simulink model "dspvorbisdec"  (Simulink 8.3)
settings: Solver=FixedStepDiscrete  SolverMode=SingleTasking  StartTime=0.0  StopTime=inf  RelTol=1e-3
model workspace (MAT data in the model file):
  oggData = [79 103 103 83 0 2 0 0 0 0 0 0 ... (70501 elements, 70501x1)]
  dspvorbisdec_OutputSampRt : num (value not decoded)
PostLoadFcn:
  | hws  = get_param(bdroot,'modelworkspace');
  | dspvorbisdec_SampRt = hws.evalin('dspvorbisdec_OutputSampRt');
  | clear hws;
StopFcn:
  | dspvorbisdec_hws = get_param(bdroot,'modelworkspace');
  | dspvorbisdec_tmp = dspvorbisdec_hws.data;
  | for i = 1:length(dspvorbisdec_tmp)
  |   if strcmp(dspvorbisdec_tmp(i).Name,'dspvorbisdec_OutputSampRt')
  |      if (dspvorbisdec_tmp(i).Value~=dspvorbisdec_SampRt)
  |         dspvorbisdec_hws.assignin('dspvorbisdec_OutputSampRt', dspvorbisdec_SampRt);
  |      end
  |   end
  | end
  | 
  | clear hws dspvorbisdec_tmp i dspvorbisdec_hws;
undefined symbols (not defined in the file or in its folder): blockSize, errordlg, uiwait, warndlg
libraries: simulink x5, dspmtrx3 x3, dspindex x2, dspsigops x1, dspxfrm3 x1, dspmisc x1, dspsnks4 x1, dspsrcs4 x1
(part 1 of 3)
CloseFcn:
  | clear dspvorbisdec_SampRt;
settings Model: FPTRunName=Active  Creator=The MathWorks Inc.  ExtModeAutoUpdateStatusClock=off
settings DataIOCC: SaveOutput=off  SignalLogging=off  SaveTime=off
settings OptimizationCC: InlineParams=on  ExpressionDepthLimit=2147483647  InitFltsAndDblsToZero=on  EfficientMapNaN2IntZero=off
settings DebuggingCC: SaveWithParameterizedLinksMsg=none  MultiTaskDSMMsg=warning  MultiTaskCondExecSysMsg=none  FcnCallInpInsideContextMsg=UseLocalSettings  StrictBusMsg=Warning
settings HardwareCC: TargetBitPerLong=64  TargetBitPerPointer=64  TargetLongLongMode=on  TargetEndianess=LittleEndian  TargetWordSize=64  TargetHWDeviceType=MATLAB Host  ProdEqTarget=off
settings SFSimCC: SFSimEnableDebug=off  SFSimOverflowDetection=off  SFSimEcho=off  SimParseCustomCode=off
settings GRTTargetCC: TargetFcnLib=ansi_tfl_tmw.mat

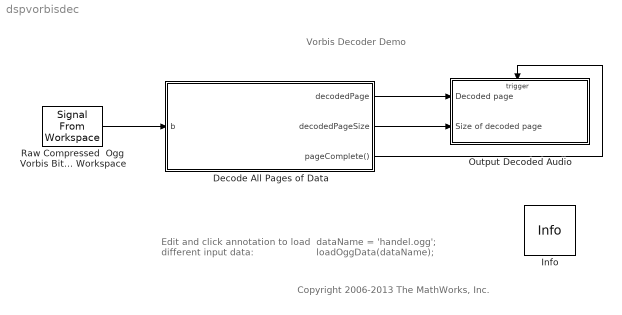
== system dspvorbisdec ==
  note: Vorbis Decoder Demo
  note: Copyright 2006-2013 The MathWorks, Inc.
  note: dataName = 'handel.ogg';
      | loadOggData(dataName);
  note: Edit and click annotation to
      | load different input data:
  Decode All Pages of Data : Stateflow chart  TreatAsAtomicUnit=on
  Info : dspmisc/Info  SystemSampleTime=-1
  Output Decoded Audio : Subsystem  TreatAsAtomicUnit=on
  Raw Compressed  Ogg Vorbis Bitstream  from Workspace : dspsrcs4/Signal From Workspace  X=oggData  Ts=1  nsamps=1  OutputAfterFinalValue=Cyclic repetition  ignoreOrWarnInputAndFrameLengths=off
  wires:
  Raw Compressed  Ogg Vorbis Bitstream  from Workspace/1 -> Decode All Pages of Data/1(b)
  Decode All Pages of Data/3(pageComplete()) -> Output Decoded Audio/Trigger
  Decode All Pages of Data/1(decodedPage) -> Output Decoded Audio/1(Decoded page)
  Decode All Pages of Data/2(decodedPageSize) -> Output Decoded Audio/2(Size of decoded page)

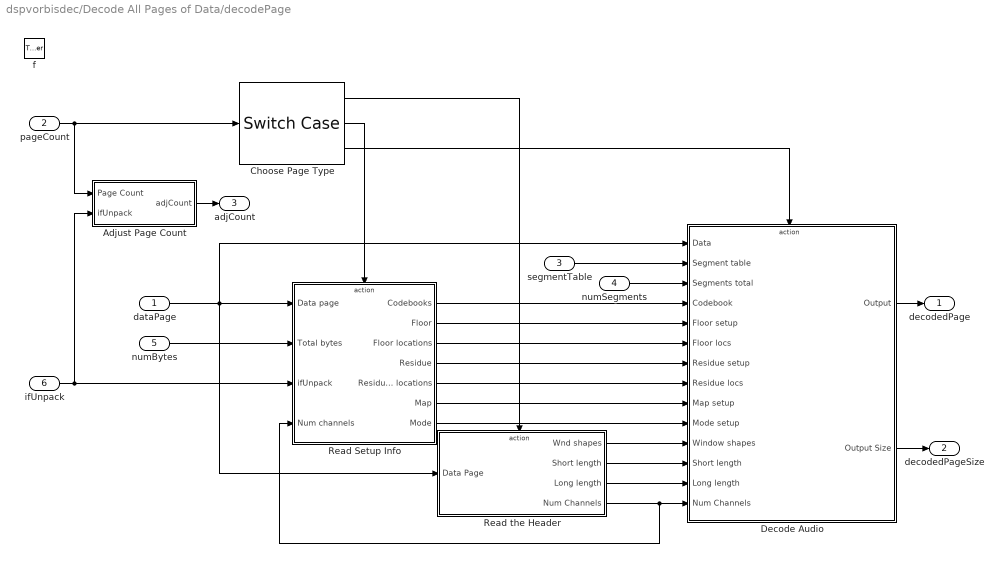
== system dspvorbisdec/Decode All Pages of Data/decodePage ==
  dataPage : Inport  OutDataTypeStr=uint8  PortDimensions=5500
  pageCount : Inport  Port=2  OutDataTypeStr=uint16  PortDimensions=1
  segmentTable : Inport  Port=3  OutDataTypeStr=uint16  PortDimensions=255
  numSegments : Inport  Port=4  OutDataTypeStr=uint16  PortDimensions=1
  numBytes : Inport  Port=5  OutDataTypeStr=uint16  PortDimensions=1
  ifUnpack : Inport  Port=6  OutDataTypeStr=boolean  PortDimensions=1
  f : TriggerPort  TriggerType=function-call
      settings: CopyFcn=Stateflow.SLINSF.SimulinkMan.removeBlockPreDeleteFcn  PreDeleteFcn=Stateflow.SLINSF.SimulinkMan.unsafePredeleteFcn
  Adjust Page Count : Subsystem
  Choose Page Type : SwitchCase  CaseConditions={1, 2}
  Decode Audio : Subsystem  TreatAsAtomicUnit=on
  Read Setup Info : Subsystem  TreatAsAtomicUnit=on
  Read the Header : Subsystem  TreatAsAtomicUnit=on
  decodedPage : Outport
  decodedPageSize : Outport  Port=2  OutputWhenDisabled=reset  InitialOutput=0
  adjCount : Outport  Port=3  OutputWhenDisabled=reset  InitialOutput=0
  wires:
  dataPage/1 -> Read the Header/1(Data Page), Decode Audio/1(Data), Read Setup Info/1(Data page)
  pageCount/1 -> Choose Page Type/1, Adjust Page Count/1(Page Count)
  Choose Page Type/1 -> Read the Header/Action
  Choose Page Type/2 -> Read Setup Info/Action
  numBytes/1 -> Read Setup Info/2(Total bytes)
  Read Setup Info/7(Mode) -> Decode Audio/10(Mode setup)
  Read Setup Info/6(Map) -> Decode Audio/9(Map setup)
  Read Setup Info/5(Residue locations) -> Decode Audio/8(Residue locs)
  Read Setup Info/4(Residue) -> Decode Audio/7(Residue setup)
  Read Setup Info/3(Floor locations) -> Decode Audio/6(Floor locs)
  Read Setup Info/2(Floor) -> Decode Audio/5(Floor setup)
  Read Setup Info/1(Codebooks) -> Decode Audio/4(Codebook)
  numSegments/1 -> Decode Audio/3(Segments total)
  segmentTable/1 -> Decode Audio/2(Segment table)
  Read the Header/1(Wnd shapes) -> Decode Audio/11(Window shapes)
  Read the Header/4(Num Channels) -> Decode Audio/14(Num Channels), Read Setup Info/4(Num channels)
  Read the Header/3(Long length) -> Decode Audio/13(Long length)
  Read the Header/2(Short length) -> Decode Audio/12(Short length)
  Decode Audio/1(Output) -> decodedPage/1
  Decode Audio/2(Output Size) -> decodedPageSize/1
  Choose Page Type/3 -> Decode Audio/Action
  ifUnpack/1 -> Read Setup Info/3(ifUnpack), Adjust Page Count/2(ifUnpack)
  Adjust Page Count/1(adjCount) -> adjCount/1

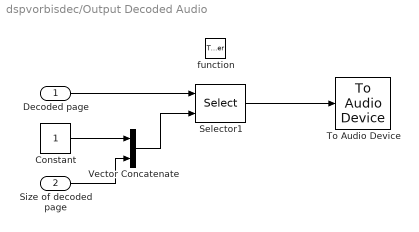
== system dspvorbisdec/Output Decoded Audio ==
  Decoded page : Inport
  Size of decoded page : Inport  Port=2
  function : TriggerPort  TriggerType=function-call
  Constant : Constant  OutDataTypeStr=int32
  Selector1 : Selector  NumberOfDimensions=2  IndexMode=Zero-based  InputPortWidth=3  IndexOptions=Starting and ending indices (port),Select all  Indices=[1 3],1  OutputSizes=32,1
  To Audio Device : dspsnks4/To Audio Device  deviceName=Default  inheritSampleRate=off  sampleRate=dspvorbisdec_OutputSampRt  deviceDatatype=Determine from input data type  autoBufferSize=on  bufferSize=1024  queueDuration=1  defaultOutputChannelMapping=on  outputChannelMapping=1
  Vector Concatenate : Concatenate
  wires:
  Size of decoded page/1 -> Vector Concatenate/2
  Selector1/1 -> To Audio Device/1
  Constant/1 -> Vector Concatenate/1
  Vector Concatenate/1 -> Selector1/2
  Decoded page/1 -> Selector1/1

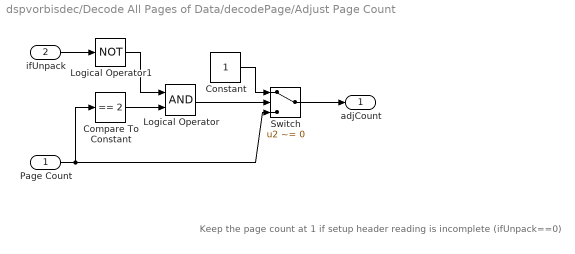
== system dspvorbisdec/Decode All Pages of Data/decodePage/Adjust Page Count ==
  note: Keep the page count at 1 if setup header reading is incomplete (ifUnpack==0)
  Page Count : Inport
  ifUnpack : Inport  Port=2
  Compare To Constant : simulink/Logic and Bit Operations/Compare To Constant  relop===  const=2  OutDataTypeStr=boolean  ZeroCross=off
  Constant : Constant  OutDataTypeStr=uint16
  Logical Operator : Logic  AllPortsSameDT=off  OutDataTypeStr=boolean
  Logical Operator1 : Logic  Operator=NOT  AllPortsSameDT=off  OutDataTypeStr=boolean
  Switch : Switch  Criteria=u2 ~= 0
  adjCount : Outport
  wires:
  Logical Operator/1 -> Switch/2
  Constant/1 -> Switch/1
  Page Count/1 -> Switch/3, Compare To Constant/1
  ifUnpack/1 -> Logical Operator1/1
  Logical Operator1/1 -> Logical Operator/1
  Compare To Constant/1 -> Logical Operator/2
  Switch/1 -> adjCount/1

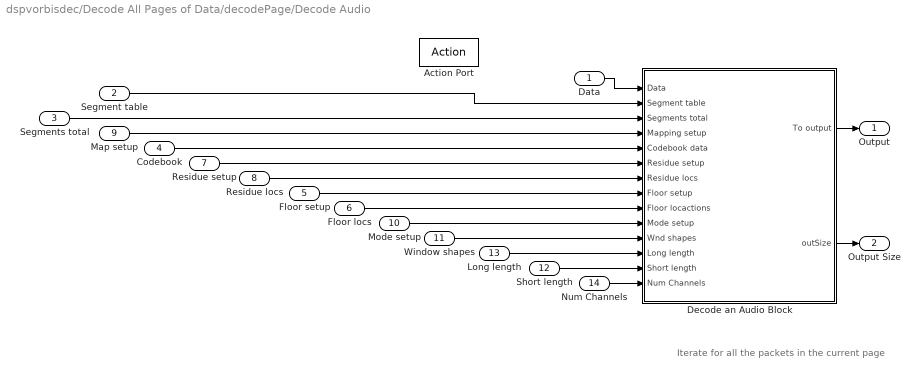
== system dspvorbisdec/Decode All Pages of Data/decodePage/Decode Audio ==
  note: Iterate for all the packets in the current page
  Data : Inport
  Segment table : Inport  Port=2
  Segments total : Inport  Port=3
  Codebook : Inport  Port=4
  Floor setup : Inport  Port=5
  Floor locs : Inport  Port=6
  Residue setup : Inport  Port=7
  Residue locs : Inport  Port=8
  Map setup : Inport  Port=9
  Mode setup : Inport  Port=10
  Window shapes : Inport  Port=11
  Short length : Inport  Port=12
  Long length : Inport  Port=13
  Num Channels : Inport  Port=14
  Action Port : ActionPort  PropagateVarSize=During execution  ActionType=default
  Decode an Audio Block : Subsystem  TreatAsAtomicUnit=on
  Output : Outport
  Output Size : Outport  Port=2  OutputWhenDisabled=reset  InitialOutput=0
  wires:
  Segment table/1 -> Decode an Audio Block/2(Segment table)
  Segments total/1 -> Decode an Audio Block/3(Segments total)
  Map setup/1 -> Decode an Audio Block/4(Mapping setup)
  Codebook/1 -> Decode an Audio Block/5(Codebook data)
  Residue setup/1 -> Decode an Audio Block/6(Residue setup)
  Residue locs/1 -> Decode an Audio Block/7(Residue locs)
  Floor setup/1 -> Decode an Audio Block/8(Floor setup)
  Floor locs/1 -> Decode an Audio Block/9(Floor locactions)
  Mode setup/1 -> Decode an Audio Block/10(Mode setup)
  Window shapes/1 -> Decode an Audio Block/11(Wnd shapes)
  Long length/1 -> Decode an Audio Block/12(Long length)
  Short length/1 -> Decode an Audio Block/13(Short length)
  Decode an Audio Block/1(To output) -> Output/1
  Decode an Audio Block/2(outSize) -> Output Size/1
  Num Channels/1 -> Decode an Audio Block/14(Num Channels)
  Data/1 -> Decode an Audio Block/1(Data)

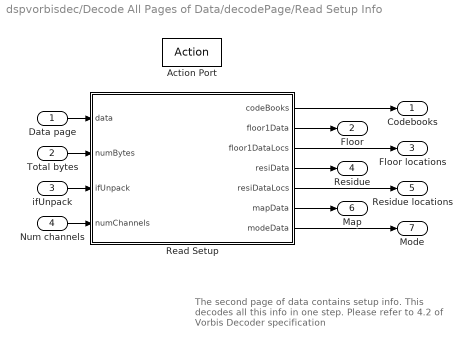
== system dspvorbisdec/Decode All Pages of Data/decodePage/Read Setup Info ==
  note: The second page of data contains
      | setup info. This decodes all this info in one step.
      | Please refer to 4.2 of Vorbis Decoder specification
  Data page : Inport
  Total bytes : Inport  Port=2
  ifUnpack : Inport  Port=3
  Num channels : Inport  Port=4
  Action Port : ActionPort  PropagateVarSize=During execution  ActionType=case
  Read Setup : MATLAB Function  TreatAsAtomicUnit=on
  Codebooks : Outport
  Floor : Outport  Port=2
  Floor locations : Outport  Port=3
  Residue : Outport  Port=4
  Residue locations : Outport  Port=5
  Map : Outport  Port=6
  Mode : Outport  Port=7
  wires:
  Data page/1 -> Read Setup/1(data)
  Total bytes/1 -> Read Setup/2(numBytes)
  Read Setup/1(codeBooks) -> Codebooks/1
  Read Setup/2(floor1Data) -> Floor/1
  Read Setup/3(floor1DataLocs) -> Floor locations/1
  Read Setup/4(resiData) -> Residue/1
  Read Setup/5(resiDataLocs) -> Residue locations/1
  Read Setup/6(mapData) -> Map/1
  Read Setup/7(modeData) -> Mode/1
  Num channels/1 -> Read Setup/4(numChannels)
  ifUnpack/1 -> Read Setup/3(ifUnpack)

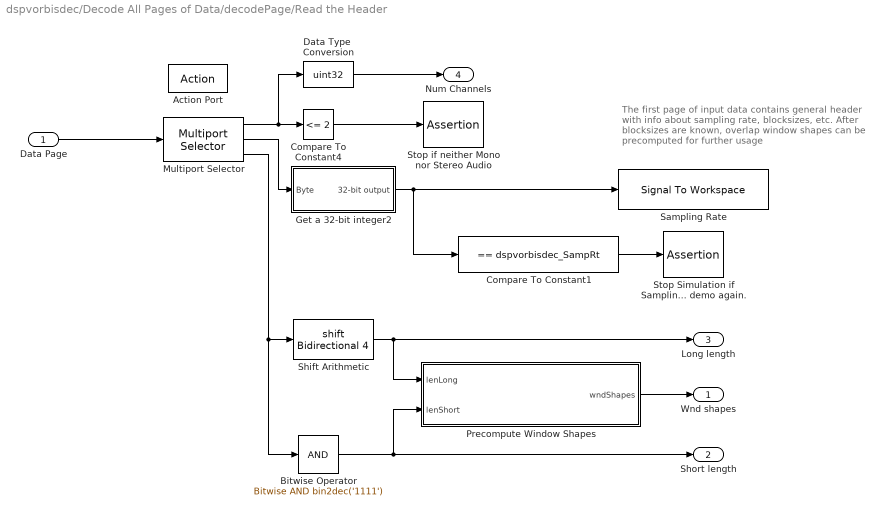
== system dspvorbisdec/Decode All Pages of Data/decodePage/Read the Header ==
  note: The first page of input data contains general header
      | with info about sampling rate, blocksizes, etc.
      | After blocksizes are known, overlap window shapes
      | can be precomputed for further usage
  Data Page : Inport
  Action Port : ActionPort  PropagateVarSize=During execution  ActionType=case
  Bitwise Operator : simulink/Logic and Bit Operations/Bitwise Operator  logicop=AND  UseBitMask=on  BitMask=bin2dec('1111')  BitMaskRealWorld=Stored Integer
  Compare To Constant1 : simulink/Logic and Bit Operations/Compare To Constant  relop===  const=dspvorbisdec_SampRt  OutDataTypeStr=boolean  ZeroCross=off
  Compare To Constant4 : simulink/Logic and Bit Operations/Compare To Constant  relop=<=  const=2  OutDataTypeStr=boolean  ZeroCross=off
  Data Type  Conversion : DataTypeConversion  OutDataTypeStr=uint32  SaturateOnIntegerOverflow=on  RndMeth=Zero
  Get a 32-bit integer2 : Subsystem
  Multiport Selector : dspindex/Multiport Selector  rowsOrCols=Rows  idxCellArray={12, 13:16, 29}  idxErrMode=Clip Index
  Precompute Window Shapes : MATLAB Function  TreatAsAtomicUnit=on
  Sampling Rate : SignalToWorkspace  VariableName=dspvorbisdec_SampRt
      settings: CopyFcn=dspblkcopystw(gcbh);  MaxDataPoints=1  Save2DSignal=3-D array (concatenate along third dimension)
  Shift Arithmetic : ArithShift  BitShiftNumber=4
  Stop Simulation if Sampling Rate is Different Than Before. Run the demo again. : Assertion  AssertionFailFcn=uiwait(warndlg('Output the sampling rate has been updated. Please stop the simulation and run the demo again.','DSP System Toolbox Demo Warning','modal'));  StopWhenAssertionFail=off
  Stop if neither Mono nor Stereo Audio : Assertion  AssertionFailFcn=uiwait(errordlg('This demo only supports monophonic or stereo audio inputs.','DSP System Toolbox Demo Error','modal'));
  Wnd shapes : Outport
  Short length : Outport  Port=2
  Long length : Outport  Port=3
  Num Channels : Outport  Port=4
  wires:
  Data Page/1 -> Multiport Selector/1
  Multiport Selector/1 -> Compare To Constant4/1, Data Type  Conversion/1
  Multiport Selector/2 -> Get a 32-bit integer2/1(Byte)
  Get a 32-bit integer2/1(32-bit output) -> Sampling Rate/1, Compare To Constant1/1
  Bitwise Operator/1 -> Precompute Window Shapes/2(lenShort), Short length/1
  Shift Arithmetic/1 -> Precompute Window Shapes/1(lenLong), Long length/1
  Precompute Window Shapes/1(wndShapes) -> Wnd shapes/1
  Multiport Selector/3 -> Shift Arithmetic/1, Bitwise Operator/1
  Compare To Constant4/1 -> Stop if neither Mono nor Stereo Audio/1
  Data Type  Conversion/1 -> Num Channels/1
  Compare To Constant1/1 -> Stop Simulation if Sampling Rate is Different Than Before. Run the demo again./1

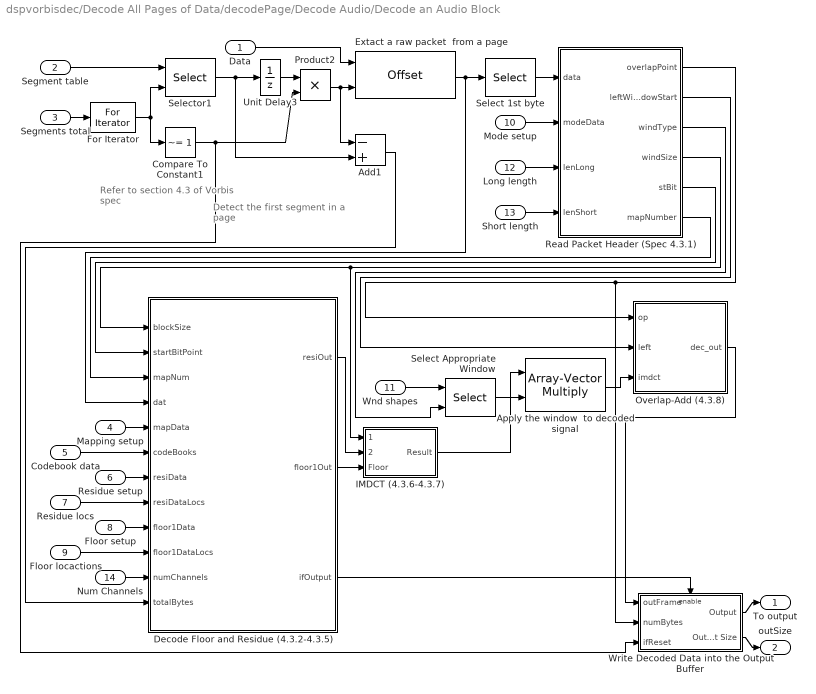
== system dspvorbisdec/Decode All Pages of Data/decodePage/Decode Audio/Decode an Audio Block ==
  note: Refer to section 4.3 of
      | Vorbis spec
  note: Detect the first
      | segment in a page
  Data : Inport
  Segment table : Inport  Port=2
  Segments total : Inport  Port=3
  Mapping setup : Inport  Port=4
  Codebook data : Inport  Port=5
  Residue setup : Inport  Port=6
  Residue locs : Inport  Port=7
  Floor setup : Inport  Port=8
  Floor locactions : Inport  Port=9
  Mode setup : Inport  Port=10
  Wnd shapes : Inport  Port=11
  Long length : Inport  Port=12
  Short length : Inport  Port=13
  Num Channels : Inport  Port=14
  Add1 : Sum  Inputs=-+
  Apply the window  to decoded signal : dspmtrx3/Array-Vector Multiply  mode=Mute  saveAsFlag=0  Dimension=1  V_Source=Input port  V_VectFromMask=[0.5 0.25]  firstCoeffSignedness=Auto  firstCoeffDataTypeStr=Inherit: Same word length as input  firstCoeffLastDataTypeStr=Inherit: Same word length as input  firstCoeffMin=[]  firstCoeffMax=[]  outputSignedness=Auto  outputDataTypeStr=Inherit: Same as product output  outputLastDataTypeStr=Inherit: Same as product output  outputMin=[]  outputMax=[]  accumSignedness=Auto  prodOutputSignedness=Auto  roundingMode=Floor  overflowMode=off
  Compare To Constant1 : simulink/Logic and Bit Operations/Compare To Constant  relop=~=  const=1  OutDataTypeStr=uint8  ZeroCross=off
  Decode Floor and Residue (4.3.2-4.3.5) : MATLAB Function  TreatAsAtomicUnit=on
  Extact a raw packet  from a page : dspsigops/Offset  mode=Remove beginning samples  numDatOffPair=1  outWidthSpec=User-defined  outWidth=2048  actionOutRange=Clip
  For Iterator : ForIterator  IterationSource=external
  IMDCT (4.3.6-4.3.7) : Subsystem
  Overlap-Add (4.3.8) : Subsystem
  Product2 : Product  OutDataTypeStr=uint16  RndMeth=Zero
  Read Packet Header (Spec 4.3.1) : MATLAB Function  TreatAsAtomicUnit=on
  Select 1st byte : Selector  InputPortWidth=2048  Indices=[1]
  Select Appropriate Window : Selector  NumberOfDimensions=2  InputPortWidth=8192  IndexOptions=Select all,Index vector (port)  Indices=1,-1
  Selector1 : Selector  InputPortWidth=255  IndexOptions=Index vector (port)  Indices=[1 3]
  Unit Delay3 : UnitDelay  SampleTime=-1
  Write Decoded Data into the Output Buffer : Subsystem  TreatAsAtomicUnit=on
  To output : Outport
  outSize : Outport  Port=2
  wires:
  Segments total/1 -> For Iterator/1
  Segment table/1 -> Selector1/1
  Unit Delay3/1 -> Product2/1
  Compare To Constant1/1 -> Product2/2, Write Decoded Data into the Output Buffer/3(ifReset)
  For Iterator/1 -> Selector1/2, Compare To Constant1/1
  Mode setup/1 -> Read Packet Header (Spec 4.3.1)/2(modeData)
  Long length/1 -> Read Packet Header (Spec 4.3.1)/3(lenLong)
  Short length/1 -> Read Packet Header (Spec 4.3.1)/4(lenShort)
  Mapping setup/1 -> Decode Floor and Residue (4.3.2-4.3.5)/5(mapData)
  Codebook data/1 -> Decode Floor and Residue (4.3.2-4.3.5)/6(codeBooks)
  Residue setup/1 -> Decode Floor and Residue (4.3.2-4.3.5)/7(resiData)
  Residue locs/1 -> Decode Floor and Residue (4.3.2-4.3.5)/8(resiDataLocs)
  Floor setup/1 -> Decode Floor and Residue (4.3.2-4.3.5)/9(floor1Data)
  Floor locactions/1 -> Decode Floor and Residue (4.3.2-4.3.5)/10(floor1DataLocs)
  Read Packet Header (Spec 4.3.1)/5(stBit) -> Decode Floor and Residue (4.3.2-4.3.5)/2(startBitPoint)
  Read Packet Header (Spec 4.3.1)/6(mapNumber) -> Decode Floor and Residue (4.3.2-4.3.5)/3(mapNum)
  Decode Floor and Residue (4.3.2-4.3.5)/2(floor1Out) -> IMDCT (4.3.6-4.3.7)/3(Floor)
  Read Packet Header (Spec 4.3.1)/4(windSize) -> Decode Floor and Residue (4.3.2-4.3.5)/1(blockSize), IMDCT (4.3.6-4.3.7)/1(Wnd len)
  Read Packet Header (Spec 4.3.1)/3(windType) -> Select Appropriate Window/2
  Read Packet Header (Spec 4.3.1)/2(leftWindowStart) -> Overlap-Add (4.3.8)/2(left)
  Read Packet Header (Spec 4.3.1)/1(overlapPoint) -> Write Decoded Data into the Output Buffer/2(numBytes), Overlap-Add (4.3.8)/1(op)
  Extact a raw packet  from a page/1 -> Select 1st byte/1, Decode Floor and Residue (4.3.2-4.3.5)/4(dat)
  Select 1st byte/1 -> Read Packet Header (Spec 4.3.1)/1(data)
  Product2/1 -> Extact a raw packet  from a page/2, Add1/1
  Data/1 -> Extact a raw packet  from a page/1
  Num Channels/1 -> Decode Floor and Residue (4.3.2-4.3.5)/11(numChannels)
  IMDCT (4.3.6-4.3.7)/1(Result) -> Apply the window  to decoded signal/1
  Add1/1 -> Decode Floor and Residue (4.3.2-4.3.5)/12(totalBytes)
  Selector1/1 -> Unit Delay3/1, Add1/2
  Write Decoded Data into the Output Buffer/1(Output) -> To output/1
  Decode Floor and Residue (4.3.2-4.3.5)/1(resiOut) -> IMDCT (4.3.6-4.3.7)/2(Residue)
  Decode Floor and Residue (4.3.2-4.3.5)/3(ifOutput) -> Write Decoded Data into the Output Buffer/Enable
  Wnd shapes/1 -> Select Appropriate Window/1
  Select Appropriate Window/1 -> Apply the window  to decoded signal/2
  Apply the window  to decoded signal/1 -> Overlap-Add (4.3.8)/3(imdct)
  Overlap-Add (4.3.8)/1(dec_out) -> Write Decoded Data into the Output Buffer/1(outFrame)
  Write Decoded Data into the Output Buffer/2(Output Size) -> outSize/1

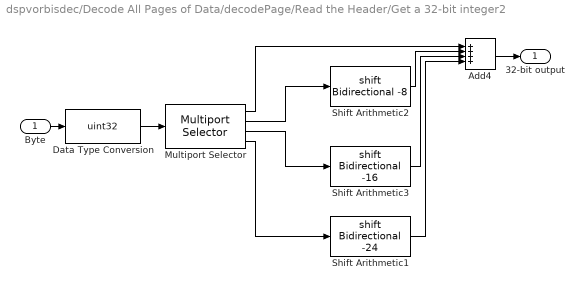
== system dspvorbisdec/Decode All Pages of Data/decodePage/Read the Header/Get a 32-bit integer2 ==
  Byte : Inport
  Add4 : Sum  Inputs=++++
  Data Type Conversion : DataTypeConversion  OutDataTypeStr=uint32  ConvertRealWorld=Stored Integer (SI)
  Multiport Selector : dspindex/Multiport Selector  rowsOrCols=Rows  idxCellArray={ 1,2,3,4 }  idxErrMode=Clip Index
  Shift Arithmetic1 : ArithShift  BitShiftNumber=-24
  Shift Arithmetic2 : ArithShift  BitShiftNumber=-8
  Shift Arithmetic3 : ArithShift  BitShiftNumber=-16
  32-bit output : Outport
  wires:
  Multiport Selector/4 -> Shift Arithmetic1/1
  Multiport Selector/1 -> Add4/1
  Data Type Conversion/1 -> Multiport Selector/1
  Multiport Selector/2 -> Shift Arithmetic2/1
  Multiport Selector/3 -> Shift Arithmetic3/1
  Add4/1 -> 32-bit output/1
  Byte/1 -> Data Type Conversion/1
  Shift Arithmetic3/1 -> Add4/3
  Shift Arithmetic2/1 -> Add4/2
  Shift Arithmetic1/1 -> Add4/4

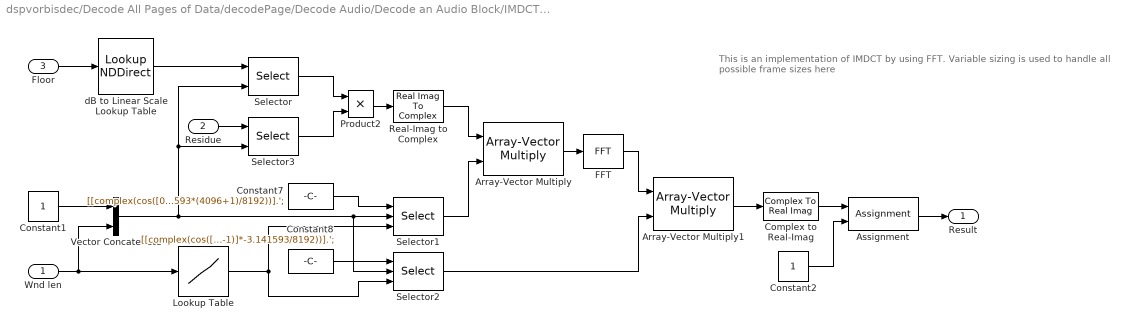
== system dspvorbisdec/Decode All Pages of Data/decodePage/Decode Audio/Decode an Audio Block/IMDCT (4.3.6-4.3.7) ==
  note: This is an implementation of IMDCT by using FFT.
      | Variable sizing is used to handle all possible frame sizes here
  Wnd len : Inport
  Residue : Inport  Port=2
  Floor : Inport  Port=3
  Array-Vector Multiply : dspmtrx3/Array-Vector Multiply  mode=Mute  saveAsFlag=0  Dimension=1  V_Source=Input port  V_VectFromMask=[0.5 0.25]  firstCoeffSignedness=Auto  firstCoeffDataTypeStr=Inherit: Same word length as input  firstCoeffLastDataTypeStr=Inherit: Same word length as input  firstCoeffMin=[]  firstCoeffMax=[]  outputSignedness=Auto  outputDataTypeStr=Inherit: Same as product output  outputLastDataTypeStr=Inherit: Same as product output  outputMin=[]  outputMax=[]  accumSignedness=Auto  prodOutputSignedness=Auto  roundingMode=Floor  overflowMode=off
  Array-Vector Multiply1 : dspmtrx3/Array-Vector Multiply  mode=Mute  saveAsFlag=0  Dimension=1  V_Source=Input port  V_VectFromMask=[0.5 0.25]  firstCoeffSignedness=Auto  firstCoeffDataTypeStr=Inherit: Same word length as input  firstCoeffLastDataTypeStr=Inherit: Same word length as input  firstCoeffMin=[]  firstCoeffMax=[]  outputSignedness=Auto  outputDataTypeStr=Inherit: Same as product output  outputLastDataTypeStr=Inherit: Same as product output  outputMin=[]  outputMax=[]  accumSignedness=Auto  prodOutputSignedness=Auto  roundingMode=Floor  overflowMode=off
  Assignment : Assignment  NumberOfDimensions=2  OutputInitialize=Specify size for each dimension in table  IndexOptions=Starting index (port),Assign all  Indices=0,1  OutputSizes=8192,2
  Complex to Real-Imag : ComplexToRealImag  Output=Real
  Constant1 : Constant  OutDataTypeStr=uint32
  Constant2 : Constant
  Constant7 : Constant  Value=[[complex(cos([0:1:(64-1)]*-3.141593*(32+1)/64),sin([0:1:(64-1)]*-3.141593*(32+1)/64)) zeros(1,8128)]; [complex(cos([0:1:(128-1)]*-3.141593*(64+1)/128),sin([0:1:(128-1)]*-3.141593*(64+1)/128)) zeros(1,8064)]; [complex(cos([0:1:(256-1)]*-3.141593*(128+1)/256),sin([0:1:(256-1)]*-3.141593*(128+1)/256)) zeros(1,7936)]; [complex(cos([0:1:(512-1)]*-3.141593*(256+1)/512),sin([0:1:(512-1)]*-3.141593*(256+1)/512)) zeros(1,7680)]; [complex(cos([0:1:(1024-1)]*-3.141593*(512+1)/1024),sin([0:1:(1024-1)]*-3.141593*(512+1)/1024)) zeros(1,7168)]; [complex(cos([0:1:(2048-1)]*-3.141593*(1024+1)/2048),sin([0:1:(2048-1)]*-3.141593*(1024+1)/2048)) zeros(1,6144)]; [complex(cos([0:1:(4096-1)]*-3.141593*(2048+1)/4096),sin([0:1:(4096-1)]*-3.141593*(2048+1)/4096)) zeros(1,4096)]; complex(cos([0:1:(8192-1)]*-3.141593*(4096+1)/8192),sin([0:1:(8192-1)]*-3.141593*(4096+1)/8192))].';  OutDataTypeStr=double
  Constant8 : Constant  Value=[[complex(cos([0:1:(64-1)]*-3.141593/64),sin([0:1:(64-1)]*-3.141593/64)) zeros(1,8128)]; [complex(cos([0:1:(128-1)]*-3.141593/128),sin([0:1:(128-1)]*-3.141593/128)) zeros(1,8064)]; [complex(cos([0:1:(256-1)]*-3.141593/256),sin([0:1:(256-1)]*-3.141593/256)) zeros(1,7936)]; [complex(cos([0:1:(512-1)]*-3.141593/512),sin([0:1:(512-1)]*-3.141593/512)) zeros(1,7680)]; [complex(cos([0:1:(1024-1)]*-3.141593/1024),sin([0:1:(1024-1)]*-3.141593/1024)) zeros(1,7168)]; [complex(cos([0:1:(2048-1)]*-3.141593/2048),sin([0:1:(2048-1)]*-3.141593/2048)) zeros(1,6144)]; [complex(cos([0:1:(4096-1)]*-3.141593/4096),sin([0:1:(4096-1)]*-3.141593/4096)) zeros(1,4096)]; complex(cos([0:1:(8192-1)]*-3.141593/8192),sin([0:1:(8192-1)]*-3.141593/8192))].';  OutDataTypeStr=double
  FFT : dspxfrm3/FFT  CompMethod=Table lookup  TableOpt=NEW  TableOptActive=Speed  BitRevOrder=off  InheritFFTLength=on  FFTLength=64  WrapInput=on  RowConvenienceOn=on  FFTImplementation=Auto  SkipNorm=off  firstCoeffDataTypeStr=Inherit: Same word length as input  firstCoeffLastDataTypeStr=Inherit: Same word length as input  outputMin=[]  outputMax=[]  roundingMode=Floor  overflowMode=off
  Lookup Table : Lookup_n-D  NumberOfTableDimensions=1  BreakpointsForDimension1=[64 128 256 512 1024 2048 4096 8192]  Table=[1 2 3 4 5 6 7 8]  ExtrapMethod=Clip  InputSameDT=on
  Product2 : Product  RndMeth=Zero
  Real-Imag to Complex : RealImagToComplex  Input=Real
  Selector : Selector  NumberOfDimensions=2  InputPortWidth=8192  IndexOptions=Starting and ending indices (port),Select all  Indices=1,1  OutputSizes=2^(blockSize+4),1
  Selector1 : Selector  NumberOfDimensions=2  InputPortWidth=8192  IndexOptions=Starting and ending indices (port),Index vector (port)  Indices=1,1  OutputSizes=2^(blockSize+4),1
  Selector2 : Selector  NumberOfDimensions=2  InputPortWidth=8192  IndexOptions=Starting and ending indices (port),Index vector (port)  Indices=1,1  OutputSizes=2^(blockSize+4),1
  Selector3 : Selector  NumberOfDimensions=2  InputPortWidth=8192  IndexOptions=Starting and ending indices (port),Select all  Indices=1,1  OutputSizes=2^(blockSize+4),1
  Vector Concatenate : Concatenate
  dB to Linear Scale Lookup Table : LookupNDDirect  NumberOfTableDimensions=1  Table=|
      | [1.0649863e-07; 1.1341951e-07; 1.2079015e-07; 1.2863978e-07; 
      | 
      |   1.3699951e-07; 1.4590251e-07; 1.5538408e-07; 1.6548181e-07; 
      | 
      |   1.7623575e-07; 1.8768855e-07; 1.9988561e-07; 2.1287530e-07; 
      | 
      |   2.2670913e-07; 2.4144197e-07; 2.5713223e-07; 2.7384213e-07; 
      | 
      |   2.9163793e-07; 3.1059021e-07; 3.3077411e-07; 3.5226968e-07; 
      | 
      |   3.7516214e-07; 3.9954229e-07; 4.2550680e-07; 4.5315863e-07; 
      | 
      |   4.8260743e-07; 5.1396998e-07; 5.4737065e-07; 5.8294187e-07; 
      | 
      |   6.2082472e-07; 6.6116941e-07; 7.0413592e-07; 7.4989464e-07; 
      | 
      |   7.9862701e-07; 8.5052630e-07; 9.0579828e-07; 9.6466216e-07; 
      | 
      |   1.0273513e-06; 1.0941144e-06; 1.1652161e-06; 1.2409384e-06; 
      | 
      |   1.3215816e-06; 1.4074654e-06; 1.4989305e-06; 1.5963394e-06; 
      | 
      |   1.7000785e-06; 1.8105592e-06; 1.9282195e-06; 2.0535261e-06; 
      | 
      |   2.1869758e-06; 2.3290978e-06; 2.4804557e-06; 2.6416497e-06; 
      | 
      |   2.8133190e-06; 2.9961443e-06; 3.1908506e-06; 3.3982101e-06; 
      | 
      |   3.6190449e-06; 3.8542308e-06; 4.1047004e-06; 4.3714470e-06; 
      | 
      |   4.6555282e-06; 4.9580707e-06; 5.2802740e-06; 5.6234160e-06; 
      | 
      |   5.9888572e-06; 6.3780469e-06; 6.7925283e-06; 7.2339451e-06; 
      | 
      |   7.7040476e-06; 8.2047000e-06; 8.7378876e-06; 9.3057248e-06; 
      | 
      |   9.9104632e-06; 1.0554501e-05; 1.1240392e-05; 1.1970856e-05; 
      | 
      |   1.2748789e-05; 1.3577278e-05; 1.4459606e-05; 1.5399272e-05; 
      | 
      |   1.6400004e-05; 1.7465768e-05; 1.8600792e-05; 1.9809576e-05; 
      | 
      |   2.1096914e-05; 2.2467911e-05; 2.3928002e-05; 2.5482978e-05; 
      | 
      |   2.7139006e-05; 2.8902651e-05; 3.0780908e-05; 3.2781225e-05; 
      | 
      |   3.4911534e-05; 3.7180282e-05; 3.9596466e-05; 4.2169667e-05; 
      | 
      |   4.4910090e-05; 4.7828601e-05; 5.0936773e-05; 5.4246931e-05; 
      | 
      |   5.7772202e-05; 6.1526565e-05; 6.5524908e-05; 6.9783085e-05; 
      | 
      |   7.4317983e-05; 7.9147585e-05; 8.4291040e-05; 8.9768747e-05; 
      | 
      |   9.5602426e-05; 0.00010181521; 0.00010843174; 0.00011547824; 
      | 
      |   0.00012298267; 0.00013097477; 0.00013948625; 0.00014855085; 
      | 
      |   0.00015820453; 0.00016848555; 0.00017943469; 0.00019109536; 
      | 
      |   0.00020351382; 0.00021673929; 0.00023082423; 0.00024582449; 
      | 
      |   0.00026179955; 0.00027881276; 0.00029693158; 0.00031622787; 
      | 
      |   0.00033677814; 0.00035866388; 0.00038197188; 0.00040679456; 
      | 
      |   0.00043323036; 0.00046138411; 0.00049136745; 0.00052329927; 
      | 
      |   0.00055730621; 0.00059352311; 0.00063209358; 0.00067317058; 
      | 
      |   0.00071691700; 0.00076350630; 0.00081312324; 0.00086596457; 
      | 
      |   0.00092223983; 0.00098217216; 0.0010459992;  0.0011139742; 
      | 
      |   0.0011863665;  0.0012634633;  0.0013455702;  0.0014330129; 
      | 
      |   0.0015261382;  0.0016253153;  0.0017309374;  0.0018434235; 
      | 
      |   0.0019632195;  0.0020908006;  0.0022266726;  0.0023713743; 
      | 
      |   0.0025254795;  0.0026895994;  0.0028643847;  0.0030505286; 
      | 
      |   0.0032487691;  0.0034598925;  0.0036847358;  0.0039241906; 
      | 
      |   0.0041792066;  0.0044507950;  0.0047400328;  0.0050480668; 
      | 
      |   0.0053761186;  0.0057254891;  0.0060975636;  0.0064938176; 
      | 
      |   0.0069158225;  0.0073652516;  0.0078438871;  0.0083536271; 
      | 
      |   0.0088964928;  0.009474637;   0.010090352;   0.010746080; 
      | 
      |   0.011444421;   0.012188144;   0.012980198;   0.013823725; 
      | 
      |   0.014722068;   0.015678791;   0.016697687;   0.017782797; 
      | 
      |   0.018938423;   0.020169149;   0.021479854;   0.022875735; 
      | 
      |   0.024362330;   0.025945531;   0.027631618;   0.029427276; 
      | 
      |   0.031339626;   0.033376252;   0.035545228;   0.037855157; 
      | 
      |   0.040315199;   0.042935108;   0.045725273;   0.048696758; 
      | 
      |   0.051861348;   0.055231591;   0.058820850;   0.062643361; 
      | 
      |   0.066714279;   0.071049749;   0.075666962;   0.080584227; 
      | 
      |   0.085821044;   0.091398179;   0.097337747;   0.10366330; 
      | 
      |   0.11039993;    0.11757434;    0.12521498;    0.13335215; 
      | 
      |   0.14201813;    0.15124727;    0.16107617;    0.17154380; 
      | 
      |   0.18269168;    0.19456402;    0.20720788;    0.22067342; 
      | 
      |   0.23501402;    0.25028656;    0.26655159;    0.28387361; 
      | 
      |   0.30232132;    0.32196786;    0.34289114;    0.36517414; 
      | 
      |   0.38890521;    0.41417847;    0.44109412;    0.46975890; 
      | 
      |   0.50028648;    0.53279791;    0.56742212;    0.60429640; 
      | 
      |   0.64356699;    0.68538959;    0.72993007;    0.77736504; 
      | 
      |   0.82788260;    0.88168307;    0.9389798;     1.00000000]
  Result : Outport
  wires:
  Product2/1 -> Real-Imag to Complex/1
  FFT/1 -> Array-Vector Multiply1/1
  Real-Imag to Complex/1 -> Array-Vector Multiply/1
  Constant1/1 -> Vector Concatenate/1
  Vector Concatenate/1 -> Selector/2, Selector3/2, Selector1/2, Selector2/2
  Selector/1 -> Product2/1
  Selector1/1 -> Array-Vector Multiply/2
  Selector2/1 -> Array-Vector Multiply1/2
  dB to Linear Scale Lookup Table/1 -> Selector/1
  Floor/1 -> dB to Linear Scale Lookup Table/1
  Wnd len/1 -> Vector Concatenate/2, Lookup Table/1
  Residue/1 -> Selector3/1
  Selector3/1 -> Product2/2
  Complex to Real-Imag/1 -> Assignment/1
  Assignment/1 -> Result/1
  Constant2/1 -> Assignment/2
  Array-Vector Multiply1/1 -> Complex to Real-Imag/1
  Array-Vector Multiply/1 -> FFT/1
  Constant7/1 -> Selector1/1
  Constant8/1 -> Selector2/1
  Lookup Table/1 -> Selector1/3, Selector2/3

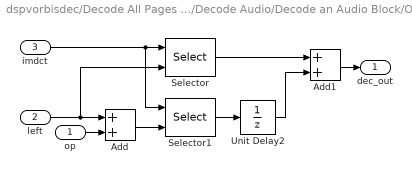
== system dspvorbisdec/Decode All Pages of Data/decodePage/Decode Audio/Decode an Audio Block/Overlap-Add (4.3.8) ==
  op : Inport
  left : Inport  Port=2
  imdct : Inport  Port=3
  Add : Sum
  Add1 : Sum
  Selector : Selector  NumberOfDimensions=2  IndexMode=Zero-based  InputPortWidth=3  IndexOptions=Starting index (port),Select all  Indices=[1 3],1  OutputSizes=4096,1
  Selector1 : Selector  NumberOfDimensions=2  IndexMode=Zero-based  InputPortWidth=3  IndexOptions=Starting index (port),Select all  Indices=[1 3],1  OutputSizes=4096,1
  Unit Delay2 : UnitDelay  SampleTime=-1
  dec_out : Outport
  wires:
  imdct/1 -> Selector/1, Selector1/1
  left/1 -> Add/1, Selector/2
  Add1/1 -> dec_out/1
  Selector1/1 -> Unit Delay2/1
  op/1 -> Add/2
  Add/1 -> Selector1/2
  Selector/1 -> Add1/1
  Unit Delay2/1 -> Add1/2

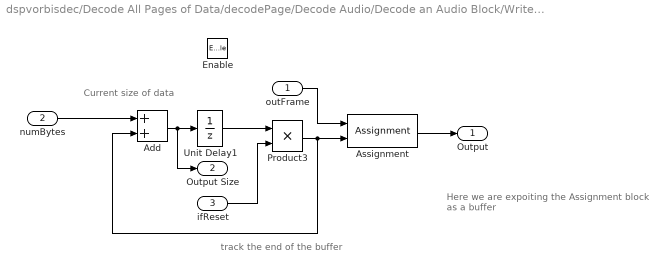
== system dspvorbisdec/Decode All Pages of Data/decodePage/Decode Audio/Decode an Audio Block/Write Decoded Data into the Output Buffer ==
  note: Here we are expoiting
      | the Assignment block as a buffer
  note: track the end of the buffer
  note: Current size of data
  outFrame : Inport
  numBytes : Inport  Port=2
  ifReset : Inport  Port=3
  Enable : EnablePort  PropagateVarSize=During execution
  Add : Sum
  Assignment : Assignment  NumberOfDimensions=2  IndexMode=Zero-based  OutputInitialize=Specify size for each dimension in table  IndexOptions=Starting index (port),Assign all  Indices=1,1  OutputSizes=55000,2
  Product3 : Product  RndMeth=Zero  OutDataTypeStr=Inherit: Same as first input
  Unit Delay1 : UnitDelay  SampleTime=-1
  Output : Outport
  Output Size : Outport  Port=2  OutputWhenDisabled=reset  InitialOutput=0
  wires:
  Product3/1 -> Add/2, Assignment/2
  Add/1 -> Unit Delay1/1, Output Size/1
  Unit Delay1/1 -> Product3/1
  Assignment/1 -> Output/1
  numBytes/1 -> Add/1
  outFrame/1 -> Assignment/1
  ifReset/1 -> Product3/2
